simulink model "observer_controls"  (R2018a)
settings: Solver=ode45  StartTime=0.0  StopTime=10  RelTol=1e-3
settings Model: Creator=HARSH  LastModifiedBy=HARSH

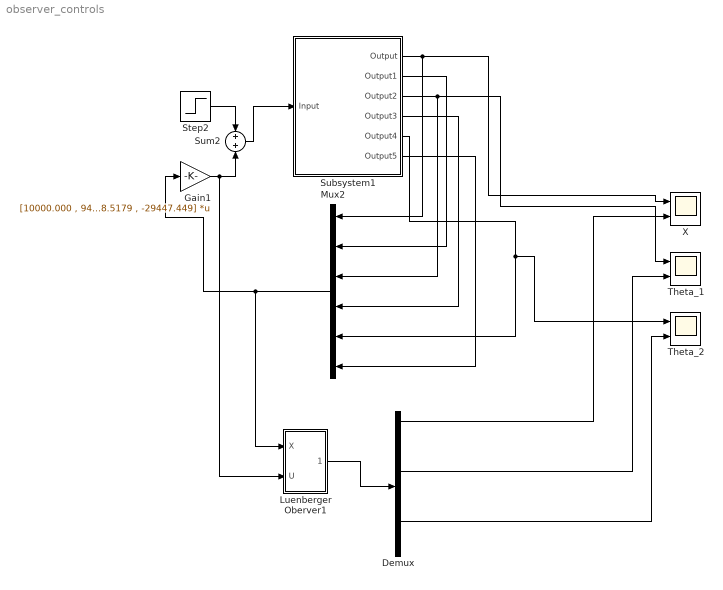
== system observer_controls ==
  Demux : Demux  Outputs=6
  Gain1 : Gain  Gain="[10000.000 , 9495.4117 ,  21169.4517 , -32255.5023 , 11278.5179 , -29447.449]"  Multiplication=Matrix(K*u)
  Luenberger Oberver1 : Subsystem
  Mux2 : Mux  Inputs=6
  Step2 : Step  After=500  SampleTime=0  VectorParams1D=off
  Subsystem1 : Subsystem
  Sum2 : Sum  Inputs=2
  Theta_1 : Scope  NumInputPorts=2
  Theta_2 : Scope  NumInputPorts=2
  X : Scope  NumInputPorts=2
  wires:
  Step2/1 -> Sum2/1
  Mux2/1 -> Luenberger Oberver1/1(X), Gain1/1
  Subsystem1/1(Output) -> X/1, Mux2/1
  Subsystem1/6(Output5) -> Mux2/6
  Sum2/1 -> Subsystem1/1(Input)
  Subsystem1/5(Output4) -> Theta_2/1, Mux2/5
  Subsystem1/3(Output2) -> Theta_1/1, Mux2/3
  Subsystem1/2(Output1) -> Mux2/2
  Subsystem1/4(Output3) -> Mux2/4
  Gain1/1 -> Luenberger Oberver1/2(U), Sum2/2
  Luenberger Oberver1/1(X_hat) -> Demux/1
  Demux/1 -> X/2
  Demux/3 -> Theta_1/2
  Demux/5 -> Theta_2/2

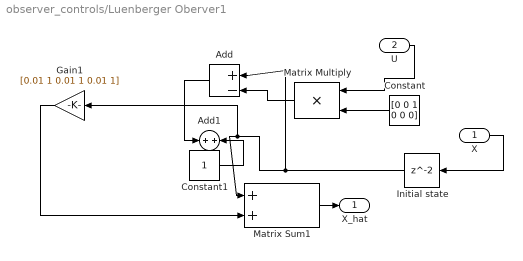
== system observer_controls/Luenberger Oberver1 ==
  X : Inport
  U : Inport  Port=2
  Add : Sum  Inputs=+|-
  Add1 : Sum
  Constant : Constant  Value=[0 0 1 0 0 0]  VectorParams1D=off
  Constant1 : Constant
  Gain1 : Gain  Gain=[0.01 1 0.01 1 0.01 1]
  Initial state : Delay  SampleTime=0.1
  Matrix Sum1 : Sum  Inputs=2
  Matrix Multiply : Product  Inputs=**  OutMin=0  OutMax=0
  X_hat : Outport
  wires:
  Matrix Sum1/1 -> X_hat/1
  X/1 -> Initial state/1
  Constant/1 -> Matrix Multiply/2
  U/1 -> Matrix Multiply/1
  Initial state/1 -> Add/1, Gain1/1, Matrix Sum1/1
  Gain1/1 -> Matrix Sum1/2
  Matrix Multiply/1 -> Add/2
  Add/1 -> Add1/1
  Constant1/1 -> Add1/2

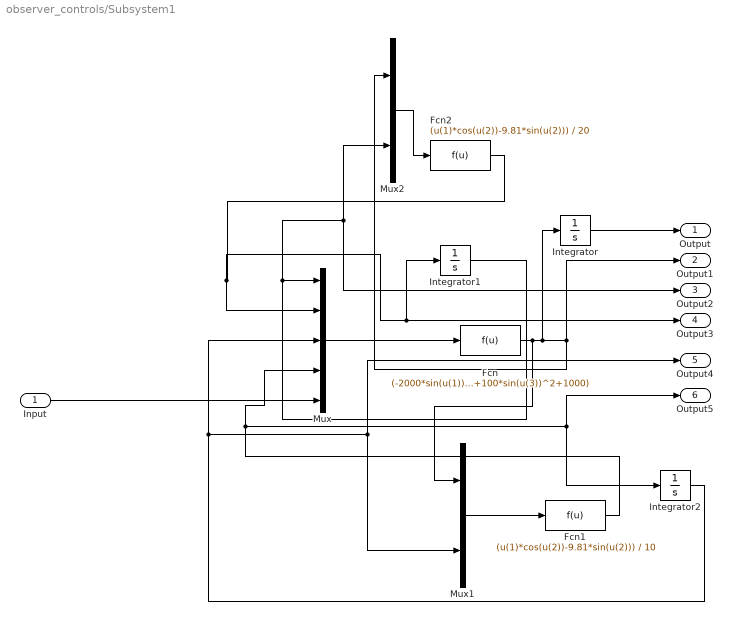
== system observer_controls/Subsystem1 ==
  Input : Inport
  Fcn : Fcn  Expr=(-2000*sin(u(1))*u(2)^2 + 1000*sin(u(3))*u(4)^2-u(5)+981*cos(u(1))*sin(u(1))+981*cos(u(3))*sin(u(3)))/(100*sin(u(1))^2+100*sin(u(3))^2+1000)
  Fcn1 : Fcn  Expr=(u(1)*cos(u(2))-9.81*sin(u(2))) / 10
  Fcn2 : Fcn  Expr=(u(1)*cos(u(2))-9.81*sin(u(2))) / 20
  Integrator : Integrator  InitialCondition=1
  Integrator1 : Integrator  InitialCondition=.2
  Integrator2 : Integrator  InitialCondition=.2
  Mux : Mux  Inputs=5
  Mux1 : Mux  Inputs=2
  Mux2 : Mux  Inputs=2
  Output : Outport
  Output1 : Outport  Port=2
  Output2 : Outport  Port=3
  Output3 : Outport  Port=4
  Output4 : Outport  Port=5
  Output5 : Outport  Port=6
  wires:
  Fcn/1 -> Mux1/1, Integrator/1, Output1/1, Mux2/1
  Input/1 -> Mux/5
  Integrator/1 -> Output/1
  Integrator2/1 -> Mux/3, Output4/1, Mux1/2
  Mux1/1 -> Fcn1/1
  Integrator1/1 -> Output2/1, Mux2/2, Mux/1
  Fcn1/1 -> Mux/4, Output5/1, Integrator2/1
  Mux2/1 -> Fcn2/1
  Fcn2/1 -> Mux/2, Output3/1, Integrator1/1
  Mux/1 -> Fcn/1
